simulink library "intertravamento"  (R2015a)
settings: Solver=ode45  SolverMode=SingleTasking  StartTime=0.0  StopTime=10.0  RelTol=1e-3
PostLoadFcn:
  | setsysloc_simulink(bdroot)
undefined symbols (not defined in the file or in its folder): docblock, getdatatypespecs, NumBits1, NumBits2, sfunxy, sigbuilder_block, slcm, SlDemoSign, Slope1, Slope2
libraries: simulink x46, sl_helperblocks x2, eml_lib x1
(part 1 of 6)
settings Model: RequirementInfo=9  FPTRunName=Active  ModifiedByFormat=The MathWorks Inc.  CovMetricSettings=d  CovSFcnEnable=off  ExtModeAutoUpdateStatusClock=off  Creator=The MathWorks Inc.  LastModifiedBy=The MathWorks Inc.
settings DataIOCC: SignalLoggingSaveFormat=ModelDataLogs
settings OptimizationCC: BlockReduction=off  BooleanDataType=off  InlineParams=on  BufferReuse=off  ExpressionDepthLimit=2147483647
settings DebuggingCC: SaveWithParameterizedLinksMsg=none  UnderspecifiedInitializationDetection=Classic  MergeDetectMultiDrivingBlocksExec=none  SignalResolutionControl=TryResolveAllWithWarning  FcnCallInpInsideContextMsg=UseLocalSettings  StateNameClashWarn=warning  StrictBusMsg=Warning
settings HardwareCC: TargetUnknown=on
settings GRTTargetCC: CombineOutputUpdateFcns=off  GRTInterface=on

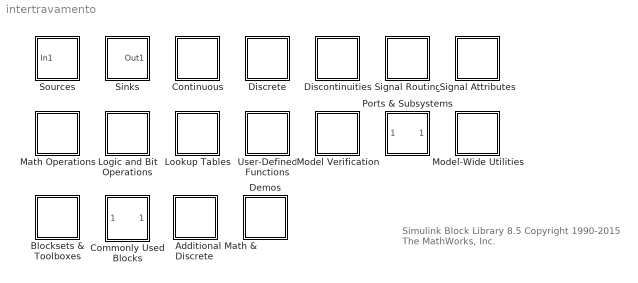
== system intertravamento ==
  note: Simulink Block Library 8.5
      | Copyright 1990-2015 The MathWorks, Inc.
  Additional Math & Discrete : Subsystem
      mask Display: image('additional_math_discrete.bmp')
  Blocksets & Toolboxes : Subsystem
      settings: OpenFcn=findblib
      mask Display: image('blocksets.bmp')
  Commonly Used Blocks : Subsystem
      mask Display: image('commonly_used.bmp')
  Continuous : Subsystem
      mask Display: image('continuous.bmp')
  Demos : Subsystem
      settings: OpenFcn=demo simulink
      mask Display:
      | image('blank_block.bmp')
      | color('darkBlue')
      | disp('Demos')
  Discontinuities : Subsystem
      mask Display: image('nonlinear.bmp')
  Discrete : Subsystem
      mask Display: image('discrete.bmp')
  Logic and Bit Operations : Subsystem
      mask Display: image('logical_bit.bmp')
  Lookup Tables : Subsystem
      mask Display: image('tables.bmp')
  Math Operations : Subsystem
      mask Display: image('math.bmp')
  Model Verification : Subsystem
      mask Display: image('assertion.bmp')
  Model-Wide Utilities : Subsystem
      mask Display:
      | image('blank_block.bmp')
      | color('darkBlue')
      | disp('Misc')
  Ports & Subsystems : Subsystem  TreatAsAtomicUnit=on
      mask Display: image('subsystems.bmp')
  Signal Attributes : Subsystem
      mask Display: image('attributes.bmp')
  Signal Routing : Subsystem
      mask Display: image('signals.bmp')
  Sinks : Subsystem
      mask Display: image('sinks.bmp')
  Sources : Subsystem
      mask Display: image('sources.bmp')
  User-Defined Functions : Subsystem
      mask Display: image('functions.bmp')

== system intertravamento/Additional Math & Discrete ==
  note: Additional Math & Discrete
  Additional Discrete : Subsystem
      mask Display: image('discrete.bmp')
  Additional Math: Increment - Decrement : Subsystem
      mask Display: image('increment_decrement.bmp')

== system intertravamento/Blocksets & Toolboxes ==

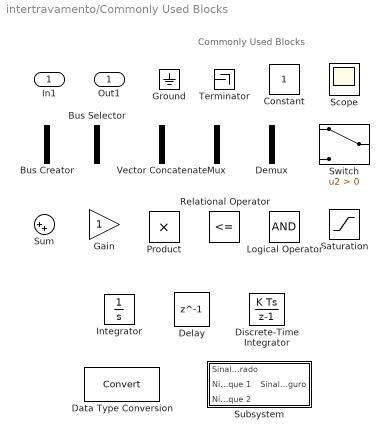
== system intertravamento/Commonly Used Blocks ==
  note: Commonly Used Blocks
  In1 : Inport
  Bus Creator : BusCreator  Inputs=2
      settings: CopyFcn=set_param(gcbh,'ShowName','off','CopyFcn','')
  Bus Selector : BusSelector  OutputSignals=signal1,signal2
      settings: CopyFcn=set_param(gcbh,'ShowName','off','CopyFcn','')
  Constant : Constant
  Data Type Conversion : DataTypeConversion
  Delay : Delay  DelayLength=1  InitialCondition=0
  Demux : Demux  Outputs=2
      settings: CopyFcn=set_param(gcbh,'ShowName','off','CopyFcn','')
  Discrete-Time Integrator : DiscreteIntegrator  InitialConditionSetting=State (most efficient)
  Gain : Gain
  Ground : Ground
  Integrator : Integrator
  Logical Operator : Logic  AllPortsSameDT=off  OutDataTypeStr=boolean
  Mux : Mux  Inputs=2
      settings: CopyFcn=set_param(gcbh,'ShowName','off','CopyFcn','')
  Product : Product
  Relational Operator : RelationalOperator  Operator=<=  OutDataTypeStr=boolean
  Saturation : Saturate
  Scope : Scope
  Subsystem : Subsystem  mask(Virtual Subsystem){}
      mask help: Simulink:masks:IOPortSubsystem_MD
      settings: CopyFcn=set_param(gcbh,'LinkStatus','none'); set_param(gcbh,'Mask','off'); set_param(gcbh,'MaskType',''); set_param(gcbh,'MaskDescription',''); set_param(gcbh,'OpenFcn',''); set_param(gcbh,'CopyFcn','')  OpenFcn=open_system(gcbh,'force')
  Sum : Sum  Inputs=|++
      settings: CopyFcn=set_param(gcbh,'ShowName','off','CopyFcn','')
  Switch : Switch  Criteria=u2 > Threshold
  Terminator : Terminator
  Vector Concatenate : Concatenate
  Out1 : Outport
